simulink model "PID_controller"  (R2020b)
settings: Solver=VariableStepAuto  StartTime=0.0  StopTime=10.0  RelTol=1e-3
undefined symbols (not defined in the file or in its folder): Kd, Ki, Kp
settings Model: DataDictionary=Cruise_control_data.sldd  Creator=JAGRUTI SHINDE  LastModifiedBy=JAGRUTI SHINDE
settings DataIOCC: SaveOutput=off  SaveTime=off

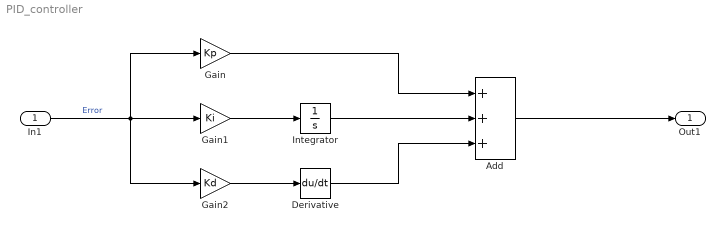
== system PID_controller ==
  In1 : Inport  OutDataTypeStr=double  PortDimensions=1  SampleTime=0
  Add : Sum  Inputs=+++
  Derivative : Derivative
  Gain : Gain  Gain=Kp
  Gain1 : Gain  Gain=Ki
  Gain2 : Gain  Gain=Kd
  Integrator : Integrator
  Out1 : Outport  OutDataTypeStr=double  PortDimensions=1  SampleTime=0
  wires:
  Add/1 -> Out1/1
  Gain/1 -> Add/1
  Gain2/1 -> Derivative/1
  Integrator/1 -> Add/2
  Gain1/1 -> Integrator/1
  Derivative/1 -> Add/3
  In1/1 -> Gain1/1, Gain2/1, Gain/1  "Error"
